simulink model "QuadcopterSimModel_Trim"  (R2018b)
settings: Solver=ode23  StartTime=0.0  StopTime=1000  FixedStep=sample_time  RelTol=1e-4  EnableMultiTasking=on
undefined symbols (not defined in the file): alt_ground, atmosphere, envir, g, wind
libraries: unit_conversions_lib x2, flight_parameters_lib x2, atmosphere_lib x1, quadcopter_lib x1
settings Model: Creator=Yannic  LastModifiedBy=yannic
settings SolverCC: ZeroCrossControl=DisableAll
settings DataIOCC: LimitDataPoints=on  ReturnWorkspaceOutputs=on
settings OptimizationCC: LifeSpan=inf
settings DebuggingCC: ReadBeforeWriteMsg=DisableAll  WriteAfterWriteMsg=DisableAll  WriteAfterReadMsg=DisableAll  MultiTaskDSMMsg=none  AllowSymbolicDim=off  LibraryContextMissingDiagnostic=none  SFUnexpectedBacktrackingDiag=warning  SFNoUnconditionalDefaultTransitionDiag=warning  SFExecutionAtInitializationDiag=none
settings ModelReferenceCC: UpdateModelReferenceTargets=IfOutOfDate  PropagateSignalLabelsOutOfModel=off
settings SFSimCC: SFSimEcho=off  SimUseLocalCustomCode=off
settings RTWCC: RTWUseLocalCustomCode=off
settings CodeAppCC: StateflowObjectComments=on
settings GRTTargetCC: TargetLangStandard=C89/C90 (ANSI)
settings ConfigComp: CovMetricSettings=dw  CovHtmlReporting=on  CovSaveCumulativeToWorkspaceVar=on  CovSaveSingleToWorkspaceVar=on  CovExternalEMLEnable=off

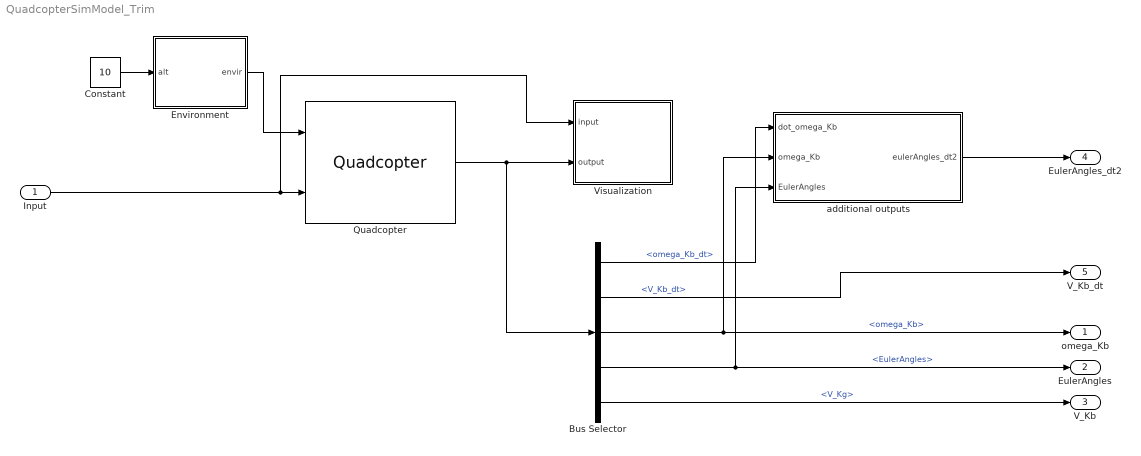
== system QuadcopterSimModel_Trim ==
  Input : Inport  PortDimensions=4
  Bus Selector : BusSelector  OutputSignals=rigidBodyBus.omega_Kb_dt,rigidBodyBus.V_Kb_dt,rigidBodyBus.omega_Kb,rigidBodyBus.EulerAngles,rigidBodyBus.V_Kg
  Constant : Constant  Value=10
  Environment : Subsystem
  Quadcopter : quadcopter_lib/Quadcopter  copter_=copter  IC_=IC  grnd_=grnd
      settings: SourceProductName=LADAC
  Visualization : Subsystem
  additional outputs : Subsystem
  omega_Kb : Outport
  EulerAngles : Outport  Port=2
  V_Kb : Outport  Port=3
  EulerAngles_dt2 : Outport  Port=4
  V_Kb_dt : Outport  Port=5
  wires:
  Bus Selector/3 -> additional outputs/2(omega_Kb), omega_Kb/1  "<omega_Kb>"
  Bus Selector/4 -> additional outputs/3(EulerAngles), EulerAngles/1  "<EulerAngles>"
  Bus Selector/5 -> V_Kb/1  "<V_Kg>"
  Environment/1(envir) -> Quadcopter/1
  Quadcopter/1 -> Visualization/2(output), Bus Selector/1
  Input/1 -> Quadcopter/2, Visualization/1(input)
  Constant/1 -> Environment/1(alt)
  additional outputs/1(eulerAngles_dt2) -> EulerAngles_dt2/1
  Bus Selector/1 -> additional outputs/1(dot_omega_Kb)  "<omega_Kb_dt>"
  Bus Selector/2 -> V_Kb_dt/1  "<V_Kb_dt>"

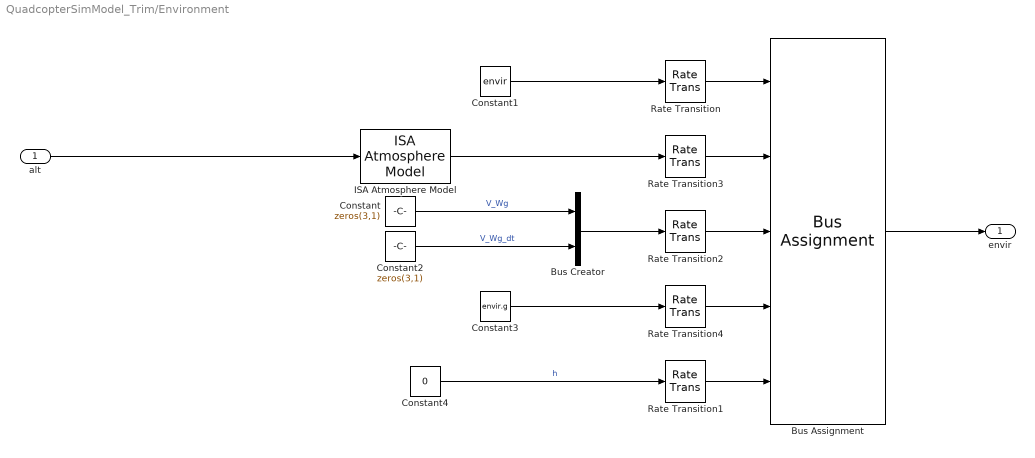
== system QuadcopterSimModel_Trim/Environment ==
  alt : Inport
  Bus Assignment : BusAssignment  AssignedSignals=atmosphere,wind,g,alt_ground
  Bus Creator : BusCreator  Inputs=2
  Constant : Constant  Value=zeros(3,1)
  Constant1 : Constant  Value=envir  OutDataTypeStr=Bus: envirBus
  Constant2 : Constant  Value=zeros(3,1)
  Constant3 : Constant  Value=envir.g
  Constant4 : Constant  Value=0
  ISA Atmosphere Model : atmosphere_lib/ISA Atmosphere Model
      settings: SourceProductName=LADAC
  Rate Transition{,1..4} (5 alike) : RateTransition
  envir : Outport
  wires:
  Constant4/1 -> Rate Transition1/1  "h"
  Rate Transition2/1 -> Bus Assignment/3
  Rate Transition3/1 -> Bus Assignment/2
  Bus Assignment/1 -> envir/1
  Rate Transition/1 -> Bus Assignment/1
  ISA Atmosphere Model/1 -> Rate Transition3/1
  Constant/1 -> Bus Creator/1  "V_Wg"
  Rate Transition1/1 -> Bus Assignment/5
  Constant1/1 -> Rate Transition/1
  alt/1 -> ISA Atmosphere Model/1
  Bus Creator/1 -> Rate Transition2/1
  Constant2/1 -> Bus Creator/2  "V_Wg_dt"
  Rate Transition4/1 -> Bus Assignment/4
  Constant3/1 -> Rate Transition4/1

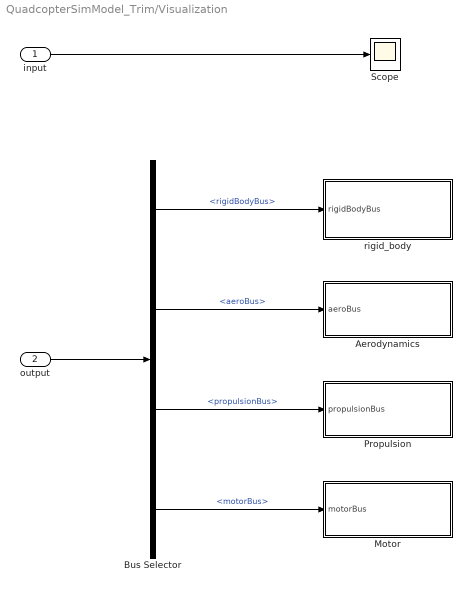
== system QuadcopterSimModel_Trim/Visualization ==
  input : Inport
  output : Inport  Port=2
  Aerodynamics : Subsystem
  Bus Selector : BusSelector  OutputSignals=rigidBodyBus,aeroBus,propulsionBus,motorBus
  Motor : Subsystem
  Propulsion : Subsystem
  Scope : Scope
  rigid_body : Subsystem
  wires:
  output/1 -> Bus Selector/1
  Bus Selector/1 -> rigid_body/1(rigidBodyBus)  "<rigidBodyBus>"
  Bus Selector/2 -> Aerodynamics/1(aeroBus)  "<aeroBus>"
  Bus Selector/3 -> Propulsion/1(propulsionBus)  "<propulsionBus>"
  Bus Selector/4 -> Motor/1(motorBus)  "<motorBus>"
  input/1 -> Scope/1

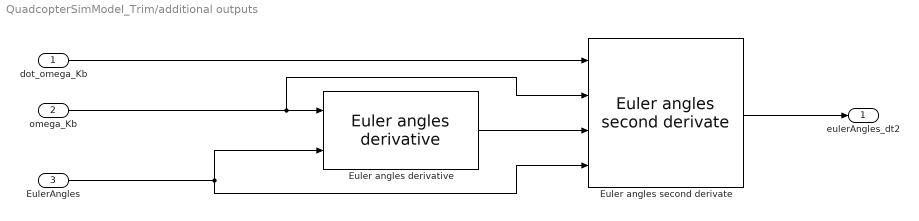
== system QuadcopterSimModel_Trim/additional outputs ==
  dot_omega_Kb : Inport
  omega_Kb : Inport  Port=2
  EulerAngles : Inport  Port=3
  Euler angles derivative : flight_parameters_lib/Euler angles derivative  SystemSampleTime=-1
      settings: SourceProductName=LADAC
  Euler angles second derivate : flight_parameters_lib/Euler angles second derivate  SystemSampleTime=-1
      settings: SourceProductName=LADAC
  eulerAngles_dt2 : Outport
  wires:
  omega_Kb/1 -> Euler angles second derivate/2, Euler angles derivative/1
  EulerAngles/1 -> Euler angles second derivate/4, Euler angles derivative/2
  Euler angles derivative/1 -> Euler angles second derivate/3
  dot_omega_Kb/1 -> Euler angles second derivate/1
  Euler angles second derivate/1 -> eulerAngles_dt2/1

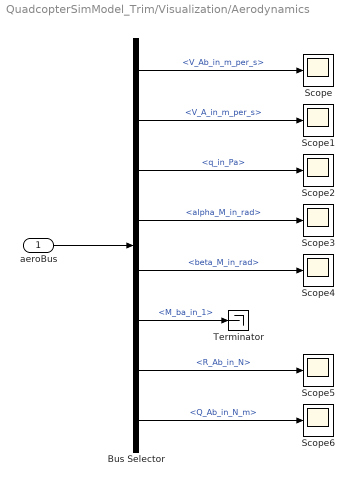
== system QuadcopterSimModel_Trim/Visualization/Aerodynamics ==
  aeroBus : Inport
  Bus Selector : BusSelector  OutputSignals=V_Ab_in_m_per_s,V_A_in_m_per_s,q_in_Pa,angles.alpha_M_in_rad,angles.beta_M_in_rad,M_ba_in_1,R_Ab_in_N,Q_Ab_in_N_m
  Scope{,1..6} (7 alike) : Scope
  Terminator : Terminator
  wires:
  aeroBus/1 -> Bus Selector/1
  Bus Selector/1 -> Scope/1  "<V_Ab_in_m_per_s>"
  Bus Selector/2 -> Scope1/1  "<V_A_in_m_per_s>"
  Bus Selector/3 -> Scope2/1  "<q_in_Pa>"
  Bus Selector/4 -> Scope3/1  "<alpha_M_in_rad>"
  Bus Selector/5 -> Scope4/1  "<beta_M_in_rad>"
  Bus Selector/6 -> Terminator/1  "<M_ba_in_1>"
  Bus Selector/7 -> Scope5/1  "<R_Ab_in_N>"
  Bus Selector/8 -> Scope6/1  "<Q_Ab_in_N_m>"

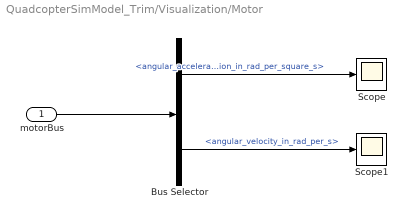
== system QuadcopterSimModel_Trim/Visualization/Motor ==
  motorBus : Inport
  Bus Selector : BusSelector  OutputSignals=angular_acceleration_in_rad_per_square_s,angular_velocity_in_rad_per_s
  Scope : Scope
  Scope1 : Scope
  wires:
  Bus Selector/1 -> Scope/1  "<angular_acceleration_in_rad_per_square_s>"
  motorBus/1 -> Bus Selector/1
  Bus Selector/2 -> Scope1/1  "<angular_velocity_in_rad_per_s>"

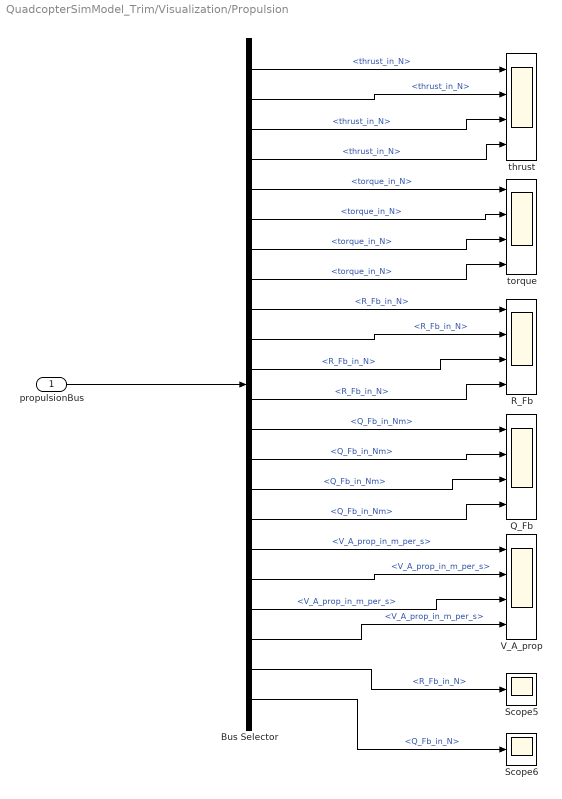
== system QuadcopterSimModel_Trim/Visualization/Propulsion ==
  propulsionBus : Inport
  Bus Selector : BusSelector  OutputSignals=propeller_1.thrust_in_N,propeller_2.thrust_in_N,propeller_3.thrust_in_N,propeller_4.thrust_in_N,propeller_1.torque_in_N,propeller_2.torque_in_N,propeller_3.torque_in_N,propeller_4.torque_in_N,propeller_1.R_Fb_in_N,propeller_2.R_Fb_in_N,propeller_3.R_Fb_in_N,propeller_4.R_Fb_in_N,propeller_1.Q_Fb_in_Nm,propeller_2.Q_Fb_in_Nm,propeller_3.Q_Fb_in_Nm,propeller_4.Q_Fb_in_Nm,propeller_1.V_A_prop_in_m_per_s,propeller_2.V_A_prop_in_m_per_s,propeller_3.V_A_prop_in_m_per_s,propeller_4.V_A_prop_in_m_per_s,R_Fb_in_N,Q_Fb_in_N
  Q_Fb : Scope  NumInputPorts=4
  R_Fb : Scope  NumInputPorts=4
  Scope5 : Scope
  Scope6 : Scope
  V_A_prop : Scope  NumInputPorts=4
  thrust : Scope  NumInputPorts=4
  torque : Scope  NumInputPorts=4
  wires:
  propulsionBus/1 -> Bus Selector/1
  Bus Selector/1 -> thrust/1  "<thrust_in_N>"
  Bus Selector/2 -> thrust/2  "<thrust_in_N>"
  Bus Selector/3 -> thrust/3  "<thrust_in_N>"
  Bus Selector/4 -> thrust/4  "<thrust_in_N>"
  Bus Selector/5 -> torque/1  "<torque_in_N>"
  Bus Selector/6 -> torque/2  "<torque_in_N>"
  Bus Selector/7 -> torque/3  "<torque_in_N>"
  Bus Selector/8 -> torque/4  "<torque_in_N>"
  Bus Selector/9 -> R_Fb/1  "<R_Fb_in_N>"
  Bus Selector/10 -> R_Fb/2  "<R_Fb_in_N>"
  Bus Selector/11 -> R_Fb/3  "<R_Fb_in_N>"
  Bus Selector/12 -> R_Fb/4  "<R_Fb_in_N>"
  Bus Selector/13 -> Q_Fb/1  "<Q_Fb_in_Nm>"
  Bus Selector/14 -> Q_Fb/2  "<Q_Fb_in_Nm>"
  Bus Selector/15 -> Q_Fb/3  "<Q_Fb_in_Nm>"
  Bus Selector/16 -> Q_Fb/4  "<Q_Fb_in_Nm>"
  Bus Selector/17 -> V_A_prop/1  "<V_A_prop_in_m_per_s>"
  Bus Selector/18 -> V_A_prop/2  "<V_A_prop_in_m_per_s>"
  Bus Selector/19 -> V_A_prop/3  "<V_A_prop_in_m_per_s>"
  Bus Selector/20 -> V_A_prop/4  "<V_A_prop_in_m_per_s>"
  Bus Selector/21 -> Scope5/1  "<R_Fb_in_N>"
  Bus Selector/22 -> Scope6/1  "<Q_Fb_in_N>"

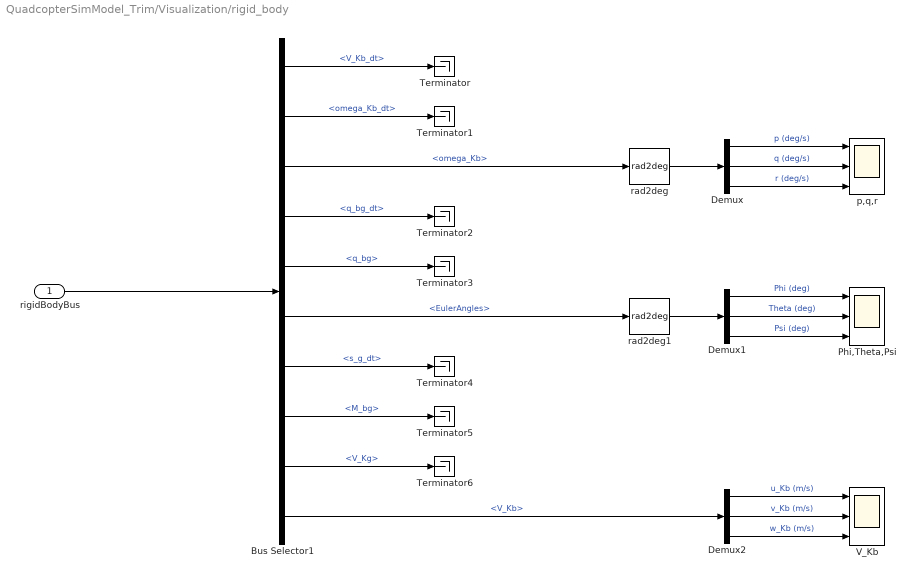
== system QuadcopterSimModel_Trim/Visualization/rigid_body ==
  rigidBodyBus : Inport
  Bus Selector1 : BusSelector  OutputSignals=V_Kb_dt,omega_Kb_dt,omega_Kb,q_bg_dt,q_bg,EulerAngles,s_g_dt,M_bg,V_Kg,V_Kb
  Demux : Demux  Outputs=3
  Demux1 : Demux  Outputs=3
  Demux2 : Demux  Outputs=3
  Phi,Theta,Psi : Scope  NumInputPorts=3
  Terminator{,1..6} (7 alike) : Terminator
  V_Kb : Scope  NumInputPorts=3
  p,q,r : Scope  NumInputPorts=3
  rad2deg : unit_conversions_lib/rad2deg
      settings: SourceProductName=LADAC
  rad2deg1 : unit_conversions_lib/rad2deg
      settings: SourceProductName=LADAC
  wires:
  Demux/1 -> p,q,r/1  "p (deg/s)"
  Demux1/2 -> Phi,Theta,Psi/2  "Theta (deg)"
  rad2deg/1 -> Demux/1
  Demux1/1 -> Phi,Theta,Psi/1  "Phi (deg)"
  Demux1/3 -> Phi,Theta,Psi/3  "Psi (deg)"
  Demux2/3 -> V_Kb/3  "w_Kb (m/s)"
  Bus Selector1/7 -> Terminator4/1  "<s_g_dt>"
  Bus Selector1/6 -> rad2deg1/1  "<EulerAngles>"
  Bus Selector1/3 -> rad2deg/1  "<omega_Kb>"
  Demux/3 -> p,q,r/3  "r (deg/s)"
  Bus Selector1/1 -> Terminator/1  "<V_Kb_dt>"
  Demux2/2 -> V_Kb/2  "v_Kb (m/s)"
  Demux/2 -> p,q,r/2  "q (deg/s)"
  rad2deg1/1 -> Demux1/1
  Bus Selector1/5 -> Terminator3/1  "<q_bg>"
  Demux2/1 -> V_Kb/1  "u_Kb (m/s)"
  Bus Selector1/10 -> Demux2/1  "<V_Kb>"
  rigidBodyBus/1 -> Bus Selector1/1
  Bus Selector1/8 -> Terminator5/1  "<M_bg>"
  Bus Selector1/4 -> Terminator2/1  "<q_bg_dt>"
  Bus Selector1/2 -> Terminator1/1  "<omega_Kb_dt>"
  Bus Selector1/9 -> Terminator6/1  "<V_Kg>"
